simulink model "lab12"  (R2017a)
settings: Solver=VariableStepAuto  StartTime=0.0  StopTime=10.0  RelTol=1e-3
InitFcn:
  | f
values from neighbouring files (symbols this model uses):
  i = 5    [f.m]
  k = -2    [f.m]
settings Model: Creator=Peter  LastModifiedBy=Peter

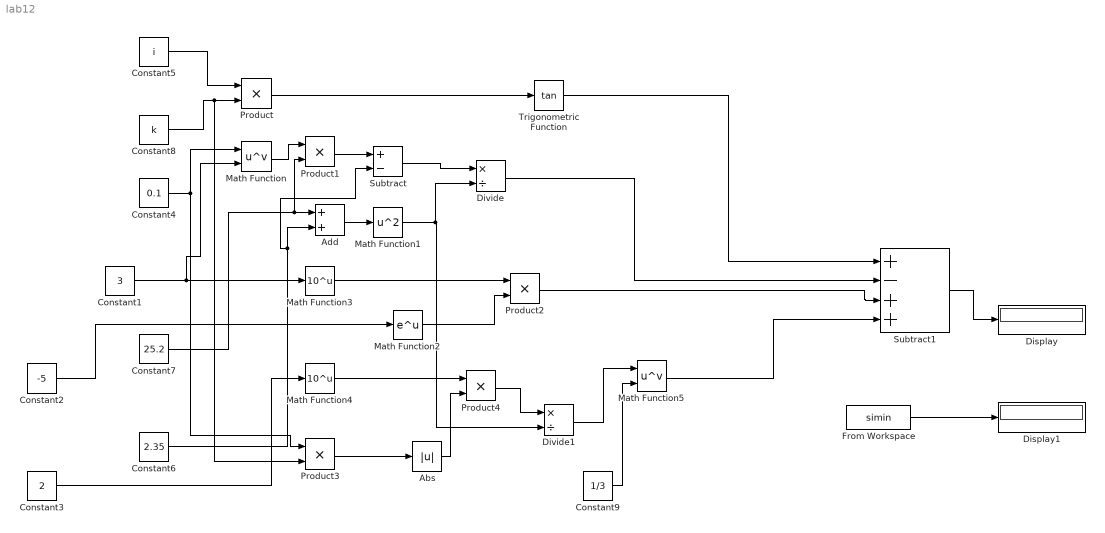
== system lab12 ==
  Abs : Abs
  Add : Sum
  Constant1 : Constant  Value=3
  Constant2 : Constant  Value=-5
  Constant3 : Constant  Value=2
  Constant4 : Constant  Value=0.1
  Constant5 : Constant  Value=i
  Constant6 : Constant  Value=2.35
  Constant7 : Constant  Value=25.2
  Constant8 : Constant  Value=k
  Constant9 : Constant  Value=1/3
  Display : Display
  Display1 : Display
  Divide : Product  Inputs=*/
  Divide1 : Product  Inputs=*/
  From Workspace : FromWorkspace  VariableName=simin  Interpolate=off  OutputAfterFinalValue=Holding final value
  Math Function : Math  Operator=pow  SaturateOnIntegerOverflow=on
  Math Function1 : Math  Operator=square  SaturateOnIntegerOverflow=on
  Math Function2 : Math  SaturateOnIntegerOverflow=on
  Math Function3 : Math  Operator=10^u  SaturateOnIntegerOverflow=on
  Math Function4 : Math  Operator=10^u  SaturateOnIntegerOverflow=on
  Math Function5 : Math  Operator=pow  SaturateOnIntegerOverflow=on
  Product{,1..4} (5 alike) : Product
  Subtract : Sum  Inputs=+-
  Subtract1 : Sum  Inputs=+-++
  Trigonometric Function : Trigonometry  Operator=tan
  wires:
  Subtract1/1 -> Display/1
  From Workspace/1 -> Display1/1
  Constant5/1 -> Product/1
  Product/1 -> Trigonometric Function/1
  Constant1/1 -> Math Function/2, Math Function3/1
  Math Function/1 -> Product1/1
  Constant7/1 -> Product1/2, Add/1
  Add/1 -> Math Function1/1
  Constant2/1 -> Math Function2/1
  Math Function3/1 -> Product2/1
  Math Function2/1 -> Product2/2
  Constant3/1 -> Math Function4/1
  Product3/1 -> Abs/1
  Constant4/1 -> Product3/1, Math Function/1
  Constant8/1 -> Product3/2, Product/2
  Math Function4/1 -> Product4/1
  Abs/1 -> Product4/2
  Product4/1 -> Divide1/1
  Math Function1/1 -> Divide1/2, Divide/2
  Divide1/1 -> Math Function5/1
  Constant9/1 -> Math Function5/2
  Trigonometric Function/1 -> Subtract1/1
  Divide/1 -> Subtract1/2
  Product2/1 -> Subtract1/3
  Math Function5/1 -> Subtract1/4
  Product1/1 -> Subtract/1
  Constant6/1 -> Subtract/2, Add/2
  Subtract/1 -> Divide/1
